simulink model "controllerNonlinear"  (R2022a)
settings: Solver=FixedStepDiscrete  StartTime=0.0  StopTime=Inf  FixedStep=50e-3  RelTol=1e-3
values from neighbouring files (symbols this model uses):
  gamma = 0.3    [simulate.m]
  k = 1    [simulate.m]
  omega_max = (pi/180)*300    (= 5.23598775598)    [simulate.m]
  u_max = 1.2    [simulate.m]
settings Model: Creator=mateu  LastModifiedBy=mateu

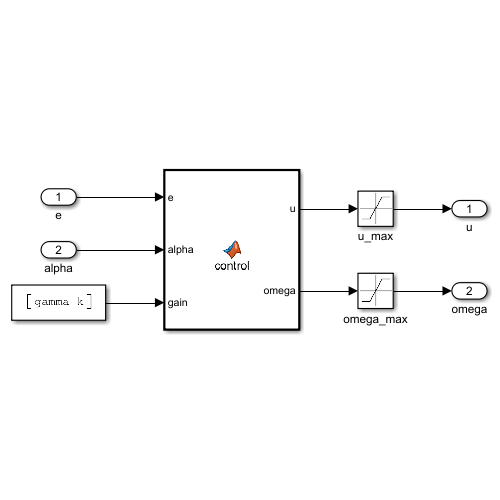
[thumbnail: Simulink's stored preview of the top-level diagram]
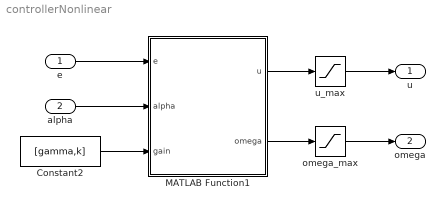
== system controllerNonlinear ==
  e : Inport
  alpha : Inport  Port=2
  Constant2 : Constant  Value=[gamma,k]
  MATLAB Function1 : MATLAB Function  TreatAsAtomicUnit=on
  omega_max : Saturate  UpperLimit=omega_max  LowerLimit=-omega_max
  u_max : Saturate  UpperLimit=u_max  LowerLimit=-u_max
  u : Outport
  omega : Outport  Port=2
  wires:
  MATLAB Function1/2(omega) -> omega_max/1
  MATLAB Function1/1(u) -> u_max/1
  u_max/1 -> u/1
  omega_max/1 -> omega/1
  alpha/1 -> MATLAB Function1/2(alpha)
  e/1 -> MATLAB Function1/1(e)
  Constant2/1 -> MATLAB Function1/3(gain)

== matlab function controllerNonlinear/MATLAB Function1 ==
  settings: updateMethod=DISCRETE  sampleTime=0.05
  data: e input; u output; alpha input; omega output; gain input
function [u,omega] = control(e,alpha,gain)

gamma = gain(1); k = gain(2);

u = gamma*e*cos(alpha);
omega = k*alpha + gamma*cos(alpha)*sin(alpha);
